simulink model "navBehavior"  (R2019b)
settings: Solver=ode23t  StartTime=0.0  StopTime=inf  RelTol=1e-3
PreLoadFcn:
  | rlMobileRobotParams;
InitFcn:
  | close all;
  | clear showPath;
model workspace (MAT data in the model file):
  mapForSim.obsMap = [0 0 0 0 0 0 0 0 0 0 0 0 ... (25000 elements, 200x125)]
  mapForSim.scaleFactor = 25
  mapForSim.simMap = robotics.BinaryOccupancyGrid
  mapForSim.simMap.Grid = [1 1 1 1 1 1 1 1 1 1 1 1 ... (25000 elements, 200x125)]
  mapForSim.simMap.LayerName = "binaryLayer"
  mapForSim.simMap.Index = matlabshared.autonomous.internal.CircularBufferIndex
  mapForSim.simMap.Index.Head = [1 1]
  mapForSim.simMap.Index.Size = [200 125]
  mapForSim.simMap.Index.NewRegions = [0 0 0 0]
  mapForSim.simMap.Index.DropEntireMap = 0
  mapForSim.simMap.Index.DropTwoRegions = [0 0]
  mapForSim.simMap.Buffer = matlabshared.autonomous.internal.CircularBuffer
  mapForSim.simMap.Buffer.ConstVal = 0
  mapForSim.simMap.Buffer.DataType = 'logical'
  mapForSim.simMap.Buffer.Index = matlabshared.autonomous.internal.CircularBufferIndex
  mapForSim.simMap.Buffer.Index.Head = [1 1]
  mapForSim.simMap.Buffer.Index.Size = [200 125]
  mapForSim.simMap.Buffer.Index.NewRegions = [0 0 0 0]
  mapForSim.simMap.Buffer.Index.DropEntireMap = 0
  mapForSim.simMap.Buffer.Index.DropTwoRegions = [0 0]
  mapForSim.simMap.Buffer.Buffer = [1 1 1 1 1 1 1 1 1 1 1 1 ... (25000 elements, 200x125)]
  mapForSim.simMap.DefaultValueInternal = 0
  mapForSim.simMap.HasParent = 0
  mapForSim.simMap.Resolution = 25
  mapForSim.simMap.GridSize = [200 125]
  mapForSim.simMap.GridOriginInLocal = [0 0]
  mapForSim.simMap.LocalOriginInWorld = [0 0]
  mapForSim.simMap.Width = 5
  mapForSim.simMap.Height = 8
  mapForSim.simMap.LocalOriginInWorldInternal = [0 0]
  occGrid = robotics.BinaryOccupancyGrid
  occGrid.Grid = [1 1 1 1 1 1 1 1 1 1 1 1 ... (25000 elements, 200x125)]
  occGrid.LayerName = "binaryLayer"
  occGrid.Index = matlabshared.autonomous.internal.CircularBufferIndex
  occGrid.Index.Head = [1 1]
  occGrid.Index.Size = [200 125]
  occGrid.Index.NewRegions = [0 0 0 0]
  occGrid.Index.DropEntireMap = 0
  occGrid.Index.DropTwoRegions = [0 0]
  occGrid.Buffer = matlabshared.autonomous.internal.CircularBuffer
  occGrid.Buffer.ConstVal = 0
  occGrid.Buffer.DataType = 'logical'
  occGrid.Buffer.Index = matlabshared.autonomous.internal.CircularBufferIndex
  occGrid.Buffer.Index.Head = [1 1]
  occGrid.Buffer.Index.Size = [200 125]
  occGrid.Buffer.Index.NewRegions = [0 0 0 0]
  occGrid.Buffer.Index.DropEntireMap = 0
  occGrid.Buffer.Index.DropTwoRegions = [0 0]
  occGrid.Buffer.Buffer = [1 1 1 1 1 1 1 1 1 1 1 1 ... (25000 elements, 200x125)]
  occGrid.DefaultValueInternal = 0
  occGrid.HasParent = 0
  occGrid.Resolution = 25
  occGrid.GridSize = [200 125]
  occGrid.GridOriginInLocal = [0 0]
  occGrid.LocalOriginInWorld = [0 0]
  occGrid.Width = 5
  occGrid.Height = 8
  occGrid.LocalOriginInWorldInternal = [0 0]
undefined symbols (not defined in the file or in its folder): goalCheckDistance, initTheta, initX, initY, map, prmConnectionDistance, prmMaxWaypoints, prmNumNodes, sampleTime
libraries: mobileRoboticsLib x3, robotalgslib x1
settings Model: Creator=josea  LastModifiedBy=scastro
settings DataIOCC: ReturnWorkspaceOutputs=off
settings DebuggingCC: UnconnectedLineMsg=none  PregeneratedLibrarySubsystemCodeDiagnostic=none  ArithmeticOperatorsInVariantConditions=warning
settings SFSimCC: SimUseLocalCustomCode=off  CustomCodeUndefinedFunction=UseInterfaceOnly
settings RTWCC: RTWUseLocalCustomCode=off
settings DiagnosticsConfigSet: SimMechanicsRigidlyBoundBlock=none
settings ExplorerConfigSet: InternalSimMechanicsExplorerSettings="<ExplorerConfiguration><canonicalview>default</canonicalview><AnimationSetting><BasePlaybackSpeed>1.0</BasePlaybackSpeed><PlaybackSpeedFactor>1.0</PlaybackSpeedFactor></AnimationSetting><TilePanel><TileInfo><Tiles Columns=\"2\" Count=\"3\" Rows=\"2\"><Column Weight=\"0.4996\"/><Column Weight=\"0.5004\"/><Row Weight=\"0.4995\"/><Row Weight=\"0.5005\"/><Tile Height=\"1\" Width=\"2\" X=\"0\" Y=\"0\"/><Tile Height=\"1\" Width=\"1\" X=\"0\" Y=\"1\"/><Tile Height=\"1\" Width=\"1\" X=\"1\" Y=\"1\"/></Tiles></TileInfo><SceneInfo><SceneViewer><BGColor><R>0.60000002384185791</R><G>0.60000002384185791</G><B>0.60000002384185791</B></BGColor><Camera><DoPerspective>off</DoPerspective><Position><X>3.21513503845026616</X><Y>-4.39133612297629217</Y><Z>3.60331941083972662</Z></Position><Center><X>0.446473736246977004</X><Y>-0.407537419322758776</Y><Z>0.493999065547941429</Z></Center><Up><X>-0.250055633923735143</X><Y>0.481736888045999345</Y><Z>0.839881986137787973</Z></Up><ViewLimDist>1</ViewLimDist><YLim>3.04422703072066758</YLim><XLim>7.99109595564175201</XLim></Camera></SceneViewer><SceneViewer><BGColor><R>0.60000002384185791</R><G>0.60000002384185791</G><B>0.60000002384185791</B></BGColor><Camera><DoPerspective>on</DoPerspective><Position><X>-0.900230893541791977</X><Y>-0.0744300644421216767</Y><Z>0.454136559277898921</Z></Position><Center><X>-1.83076580855623683</X><Y>-0.205300204269928455</Y><Z>0.112116415952230264</Z></Center><Up><X>-0.338687011010687988</X><Y>-0.047632835451577496</Y><Z>0.939692620785908428</Z></Up><ViewLimDist>1</ViewLimDist><YLim>0.466307658154998583</YLim><XLim>0.604541153655492214</XLim></Camera></SceneViewer><SceneViewer><BGColor><R>0.60000002384185791</R><G>0.60000002384185791</G><B>0.60000002384185791</B></BGColor><Camera><DoPerspective>off</DoPerspective><Position><X>-0.126032215770511102</X><Y>-0.027243386375953943</Y><Z>6.53261199512664703</Z></Position><Center><X>-0.126032215770511102</X><Y>-0.027243386375953943</Y><Z>0.127156752764657099</Z></Center><Up><X>0</X><Y>1</Y><Z>-0</Z></Up><ViewLimDist>1</ViewLimDist><YLim>4.0594907565083922</YLim><XLim>5.27894252526190133</XLim></Camera></SceneViewer></SceneInfo></TilePanel><MechEditorPanel><Cameras><Camera><Id>Camera1</Id><Value><Name>RobotView</Name><NativeCamera><PositionTrackingFeature>Obstacle_Environment.Robot.Body.RobotCamera.F</PositionTrackingFeature><CenterTrackingFeature>Obstacle_Environment.Robot.Body.RobotCamera.F</CenterTrackingFeature><UpVectorTrackingFeature>Obstacle_Environment.Robot.Body.RobotCamera.F</UpVectorTrackingFeature><CenterTrackingOrigin>off</CenterTrackingOrigin><CenterTrackingDirection>+X</CenterTrackingDirection><UpVectorTrackingDirection>+Z</UpVectorTrackingDirection></NativeCamera></Value></Camera></Cameras><GfxPanelCameraMap><MapElement CameraMLId=\"Camera1\" GfxPanelIndex=\"1\"/></GfxPanelCameraMap><VideoCreator><PlaybackSpeedRatio>1.0</PlaybackSpeedRatio><FrameRate>30</FrameRate><VideoFormat>Motion JPEG AVI</VideoFormat><FrameSize>auto</FrameSize></VideoCreator></MechEditorPanel></ExplorerConfiguration>"

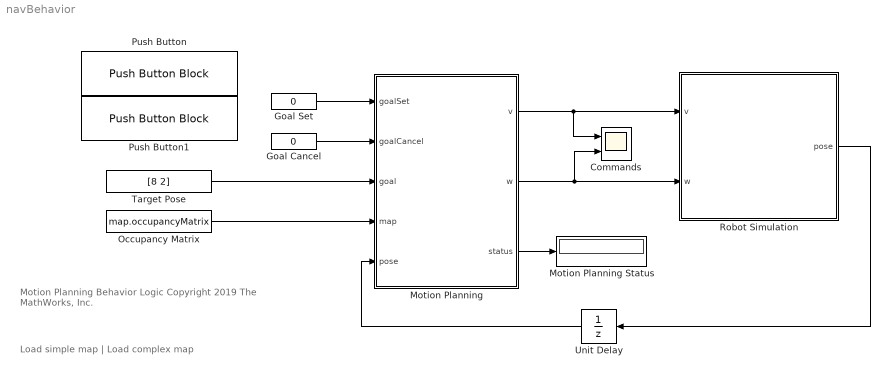
== system navBehavior ==
  note: Load simple map | Load complex map
  note: Motion Planning Behavior Logic
      | Copyright 2019 The MathWorks, Inc.
  Commands : Scope  NumInputPorts=2
  Goal Cancel : Constant  Value=0
  Goal Set : Constant  Value=0
  Motion Planning : Stateflow chart  BlockKeywords=__PRM__SERIALIZED__DATA__:Stateflow Chart,Stateflow Diagram  TreatAsAtomicUnit=on
  Motion Planning Status : Display
  Occupancy Matrix : Constant  Value=map.occupancyMatrix
  Push Button : PushButtonBlock  ButtonText=Set Nav Goal
  Push Button1 : PushButtonBlock  ButtonText=Cancel Nav Goal
  Robot Simulation : Subsystem
  Target Pose : Constant  Value=[8 2]
  Unit Delay : UnitDelay  InitialCondition=[initX;initY;initTheta]  SampleTime=-1  HasFrameUpgradeWarning=on
  wires:
  Target Pose/1 -> Motion Planning/3(goal)
  Robot Simulation/1(pose) -> Unit Delay/1
  Occupancy Matrix/1 -> Motion Planning/4(map)
  Motion Planning/1(v) -> Commands/1, Robot Simulation/1(v)
  Motion Planning/2(w) -> Robot Simulation/2(w), Commands/2
  Goal Set/1 -> Motion Planning/1(goalSet)
  Unit Delay/1 -> Motion Planning/5(pose)
  Motion Planning/3(status) -> Motion Planning Status/1
  Goal Cancel/1 -> Motion Planning/2(goalCancel)

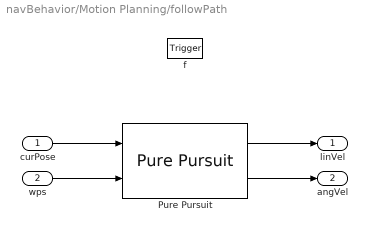
== system navBehavior/Motion Planning/followPath ==
  curPose : Inport  OutDataTypeStr=double  PortDimensions=3
  wps : Inport  Port=2  OutDataTypeStr=double  PortDimensions=[prmMaxWaypoints 2]
      settings: VarSizeSig=Yes
  f : TriggerPort  TriggerType=function-call  VariantControl=(inherit)
      settings: CopyFcn=Stateflow.SLINSF.SimulinkMan.removeBlockPreDeleteFcn  PreDeleteFcn=Stateflow.SLINSF.SimulinkMan.unsafePredeleteFcn
  Pure Pursuit : robotalgslib/Pure Pursuit  DesiredLinearVelocity=followerLinSpeed  MaxAngularVelocity=followerMaxAngSpeed  LookaheadDistance=followerLookaheadDistance  TargetDirPort=off  SimulateUsing=Interpreted execution
      settings: SourceProductName=Robotics System Toolbox  SourceProductBaseCode=RO
  linVel : Outport
  angVel : Outport  Port=2
  wires:
  curPose/1 -> Pure Pursuit/1
  wps/1 -> Pure Pursuit/2
  Pure Pursuit/1 -> linVel/1
  Pure Pursuit/2 -> angVel/1

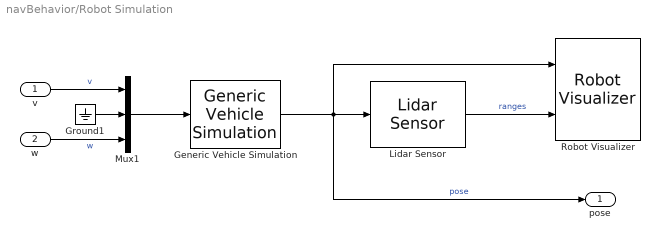
== system navBehavior/Robot Simulation ==
  v : Inport
  w : Inport  Port=2
  Generic Vehicle Simulation : mobileRoboticsLib/Utilities/Generic Vehicle Simulation  initX=initX  initY=initY  initAngle=initTheta  Ts=sampleTime
      settings: SourceProductName=Mobile Robotics Simulation Library
  Ground1 : Ground
  Lidar Sensor : mobileRoboticsLib/Environments/Lidar Sensor  mapName=map  sensorOffset=[ 0 0 ]  scanAngles=scanAngles  maxRange=maxRange
      settings: SourceProductName=Ground Vehicles Library
  Mux1 : Mux  Inputs=3
  Robot Visualizer : mobileRoboticsLib/Environments/Robot Visualizer  Priority=99  robotRadius=robotRadius  mapName=map  showTrajectory=on  hasWaypoints=off  hasLidar=on  sensorOffset=[ 0 0 ]  scanAngles=scanAngles  hasObjDetector=off  objDetectorOffset=[ 0, 0 ]  objDetectorAngle=0  objDetectorFOV=pi/4  objDetectorMaxRange=5  objectColors=[ 1, 0, 0; 0, 1, 0; 0, 0, 1 ]  objectMarkers='s'
      settings: SourceProductName=Ground Vehicles Library
  pose : Outport  VectorParamsAs1DForOutWhenUnconnected=off
  wires:
  Generic Vehicle Simulation/1 -> Lidar Sensor/1, pose/1, Robot Visualizer/1  "pose"
  Lidar Sensor/1 -> Robot Visualizer/2  "ranges"
  Ground1/1 -> Mux1/2
  w/1 -> Mux1/3  "w"
  v/1 -> Mux1/1  "v"
  Mux1/1 -> Generic Vehicle Simulation/1

== stateflow chart navBehavior/Motion Planning ==
  settings: updateMethod=DISCRETE  sampleTime=sampleTime
  state ExecuteMotionPlan
    (default) -> (junction 45) : {pathFound = false;}
    ExecuteMotionPlan -> (junction 45) [order 1]
    (junction 45) -> (junction 48) [order 1] : [pathFound]
    (junction 45) -> (junction 52) [order 2] : % Plan a path
        | {
        | [waypoints,pathFound] = ...
        | computePath(goal,pose,map);
        | }
    (junction 48) -> (junction 50) : % If a path exists, follow it
        | {
        | [v,w] = followPath(pose,waypoints);
        | status = MotionPlanning.FOLLOWING;
        | }
    (junction 50) -> (junction 52)
  state Standby
    en:
    v = 0;
    w = 0;
  state done = isGoalReached [function]
    (default) -> (junction 30) : {
        | dist = sqrt((goal(1)-pose(1))^2 + (goal(2)-pose(2))^2);
        | done = (dist <= goalCheckDistance);
        | }
  state [linVel,angVel] = followPath(curPose,wps) [function]
  (default) -> Standby
  Standby -> ExecuteMotionPlan : [hasChangedTo(goalSet,true)]
  ExecuteMotionPlan -> Standby [order 1] : % Goal is successfully reached
      | [isGoalReached]
      | {status = MotionPlanning.SUCCESS;}
  ExecuteMotionPlan -> Standby [order 2] : % User cancels motion planning
      | [hasChangedTo(goalCancel,true)]
      | {status = MotionPlanning.CANCELLED;}
  ExecuteMotionPlan -> Standby [order 3] : % Exit if path planning fails multiple times
      | [after(10,tick) && ~pathFound]
      | {status = MotionPlanning.FAILED;}
  data: done function_output; wps function_output; tgtPose function_input; curPose function_input; occMat function_input; found function_output; curPose function_input double size=3; wps function_input double size=[prmMaxWaypoints 2]; linVel function_output; angVel function_output; goalSet input; goalCancel input; v output; w output; goal input; map input; pose input; waypoints local size=[prmMaxWaypoints 2]; status output =MotionPlanning.UNASSIGNED; pathFound local; prmConnectionDistance parameter; prmNumNodes parameter; goalCheckDistance parameter
  function [wps,found] = computePath(tgtPose,curPose,occMat):
    | function [wps,found] = computePath(tgtPose,curPose,occMat)
    | 
    | % Initialize path planner on initialization
    | coder.extrinsic('showPath')
    | persistent planner firstTime
    | if isempty(planner)
    |     occMap = occupancyMap(occMat,2);
    |     inflate(occMap,0.2); % Inflate since there is no obstacle avoidance
    |     planner = mobileRobotPRM(occMap);
    |     planner.ConnectionDistance = prmConnectionDistance;
    |     planner.NumNodes = prmNumNodes;
    |     firstTime = true;
    | end
    | 
    | % Validate the input
    | found = false;
    | if (tgtPose(1) >= planner.Map.XWorldLimits(1)) && (tgtPose(1) <= planner.Map.XWorldLimits(2)) && ...
    |         (tgtPose(2) >= planner.Map.YWorldLimits(1)) && (tgtPose(2) <= planner.Map.YWorldLimits(2)) && ...
    |         (~checkOccupancy(planner.Map,[tgtPose(1) tgtPose(2)]))
    |     
    |     % If this is not the first time using the PRM, but the previous path
    |     % failed, then increase the number of nodes in the PRM and try again.
    |     if ~firstTime
    |         planner.NumNodes = planner.NumNodes + prmNumNodes;
    |     end
    |     
    |     % Find a path given start and end positions
    |     wps = findpath(planner,[curPose(1) curPose(2)],[tgtPose(1) tgtPose(2)]);
    |     
    |     % Path is successfully found if the output of "findpath" is non-empty
    |     if ~isempty(wps)
    |         found = true;
    |         planner.NumNodes = prmNumNodes;
    |         showPath(wps);
    |     else
    |         firstTime = false;
    |     end
    | else
    |     wps = [];  
    | end
